simulink model "room1"  (R2021a)
settings: Solver=FixedStepAuto  StartTime=0.0  StopTime=10.0  RelTol=1e-3  EnableMultiTasking=on
libraries: dspmtrx3 x6, simulink x2
settings Model: DataDictionary=worldDD.sldd  SILPILModeSetting=veronly  ExtModeTrigDuration=2  Creator=Koorosh  LastModifiedBy=Koorosh
settings OptimizationCC: EnhancedBackFolding=on  PassReuseOutputArgsAs=Individual arguments  ZeroExternalMemoryAtStartup=off  ZeroInternalMemoryAtStartup=off  MaxStackSize=64  OptimizeBlockOrder=speed  DifferentSizesBufferReuse=on  OptimizationCustomize=off  EfficientTunableParamExpr=on
settings DebuggingCC: ParameterTunabilityLossMsg=error
settings HardwareCC: ProdBitPerInt=16  ProdBitPerPointer=16  ProdBitPerSizeT=16  ProdBitPerPtrDiffT=16  ProdLargestAtomicFloat=None  ProdWordSize=8  ProdHWDeviceType=Atmel->AVR
settings SFSimCC: MATLABDynamicMemAlloc=off
settings RTWCC: SystemTargetFile=ert.tlc  HardwareBoard=Arduino Uno  TemplateMakefile=ert_default_tmf  Toolchain=Arduino AVR  BuildConfiguration=Faster Runs
settings CodeAppCC: ForceParamTrailComments=on  IgnoreCustomStorageClasses=off  OperatorAnnotations=on  SimulinkDataObjDesc=on  SFDataObjDesc=on  InsertBlockDesc=on
settings ERTTargetCC: SupportContinuousTime=on  SupportVariableSizeSignals=on  ExtModeStaticAllocSize=250

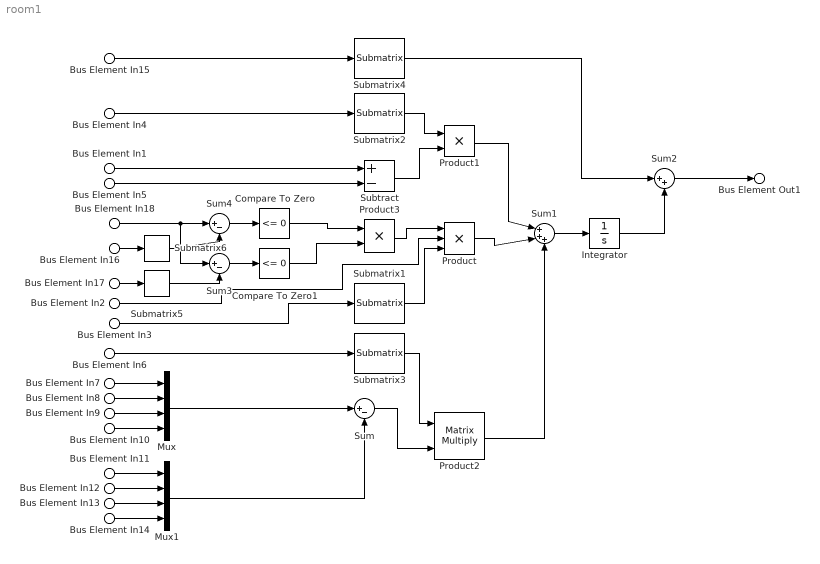
== system room1 ==
  Bus Element In1 : Inport  PortName=X  Element=u
  Bus Element In{5,7,11..14,18} (7 alike) : Inport  PortName=X  Element=x1
  Bus Element In8 : Inport  PortName=X  Element=x2
  Bus Element In9 : Inport  PortName=X  Element=x3
  Bus Element In10 : Inport  PortName=X  Element=x4
  Bus Element In2 : Inport  Port=2  PortName=H  Element=h1
  Bus Element In6 : Inport  Port=3  PortName=C  Element=A
  Bus Element In4 : Inport  Port=3  PortName=C  Element=b
  Bus Element In3 : Inport  Port=3  PortName=C  Element=c
  Bus Element In15 : Inport  Port=3  PortName=C  Element=x0
  Bus Element In17 : Inport  Port=3  PortName=C  Element=off
  Bus Element In16 : Inport  Port=3  PortName=C  Element=on
  Compare To Zero : simulink/Logic and Bit Operations/Compare To Zero  relop=<=  OutDataTypeStr=uint8
  Compare To Zero1 : simulink/Logic and Bit Operations/Compare To Zero  relop=<=  OutDataTypeStr=uint8
  Integrator : Integrator
  Mux : Mux
  Mux1 : Mux
  Product : Product  Inputs=3
  Product1 : Product
  Product2 : Product  Multiplication=Matrix(*)
  Product3 : Product
  Submatrix{1..2,4..6} (5 alike) : dspmtrx3/Submatrix  RowSpan=One row  RowStartMode=Index  RowStartIndex=1  RowEndMode=Last  RowEndIndex=1  ColSpan=One column  ColStartMode=First  ColStartIndex=1  ColEndMode=Last  ColEndIndex=1
  Submatrix3 : dspmtrx3/Submatrix  RowSpan=One row  RowStartMode=Index  RowStartIndex=1  RowEndMode=Last  RowEndIndex=1  ColSpan=All columns  ColStartMode=First  ColStartIndex=1  ColEndMode=Last  ColEndIndex=1
  Subtract : Sum  Inputs=+-
  Sum : Sum  Inputs=|+-
  Sum1 : Sum  Inputs=|+++
  Sum2 : Sum  Inputs=|++
  Sum3 : Sum  Inputs=|+-
  Sum4 : Sum  Inputs=|+-
  Bus Element Out1 : Outport  PortName=x1
  wires:
  Bus Element In3/1 -> Submatrix1/1
  Bus Element In4/1 -> Submatrix2/1
  Bus Element In1/1 -> Subtract/1
  Bus Element In5/1 -> Subtract/2
  Submatrix2/1 -> Product1/1
  Subtract/1 -> Product1/2
  Bus Element In6/1 -> Submatrix3/1
  Bus Element In7/1 -> Mux/1
  Bus Element In8/1 -> Mux/2
  Bus Element In9/1 -> Mux/3
  Bus Element In10/1 -> Mux/4
  Bus Element In11/1 -> Mux1/1
  Bus Element In12/1 -> Mux1/2
  Bus Element In13/1 -> Mux1/3
  Bus Element In14/1 -> Mux1/4
  Mux/1 -> Sum/1
  Mux1/1 -> Sum/2
  Submatrix3/1 -> Product2/1
  Sum/1 -> Product2/2
  Product1/1 -> Sum1/1
  Product/1 -> Sum1/2
  Product2/1 -> Sum1/3
  Sum1/1 -> Integrator/1
  Bus Element In15/1 -> Submatrix4/1
  Integrator/1 -> Sum2/2
  Submatrix4/1 -> Sum2/1
  Sum2/1 -> Bus Element Out1/1
  Bus Element In17/1 -> Submatrix5/1
  Bus Element In16/1 -> Submatrix6/1
  Submatrix5/1 -> Sum3/2
  Submatrix6/1 -> Sum4/2
  Sum4/1 -> Compare To Zero/1
  Sum3/1 -> Compare To Zero1/1
  Product3/1 -> Product/1
  Submatrix1/1 -> Product/3
  Bus Element In2/1 -> Product/2
  Bus Element In18/1 -> Sum3/1, Sum4/1
  Compare To Zero1/1 -> Product3/2
  Compare To Zero/1 -> Product3/1
